simulink model "amstepsize"  (Simulink 4.00)
settings: Solver=ode45  StartTime=0.0  StopTime=1  MaxStep=.01  RelTol=1e-3
undefined symbols (not defined in the file): slcm
libraries: commanapbnd2 x1
settings Model: LastModifiedBy=agaltman  InitialStep=.01  BlockReductionOpt=off

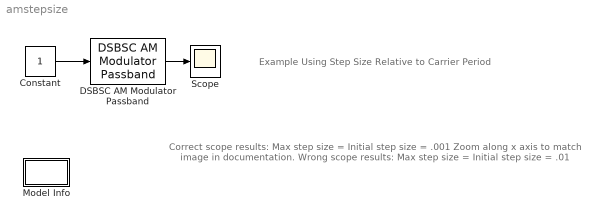
== system amstepsize ==
  note: Example Using Step Size
      | Relative to Carrier Period
  note: Correct scope results:
      | Max step size = Initial step size = .001
      | Zoom along x axis to match
      | image in documentation.
      |
      | Wrong scope results:
      | Max step size = Initial step size = .01
  Constant : Constant  Value=1
  DSBSC AM Modulator Passband : commanapbnd2/DSBSC AM Modulator Passband  Fc=100  Ph=pi/2
  Model Info : Subsystem  LoadFcn=slcm LoadBlock;  InitFcn=slcm('UpdateAllCMBlocksInThisModelInit')  mask(CMBlock){InitialSaveTempField=, InitialBlockCM=none, BlockCM=none, Frame=on, SaveTempField=, DisplayStringWithTags=Info, MaskDisplayString=Info, HorizontalTextAlignment=Center, LeftAlignmentValue=0.5, SourceBlockDiagram=amstepsize, TagMaxNumber=20, CMTag1=, CMTag2=, CMTag3=, CMTag4=, CMTag5=, CMTag6=, CMTag7=, CMTag8=, CMTag9=, CMTag10=, CMTag11=, CMTag12=, CMTag13=, CMTag14=, CMTag15=, CMTag16=, CMTag17=, CMTag18=, CMTag19=, CMTag20=}
      mask help: This block allows revision control information to be displayed within the model.
      settings: CopyFcn=slcm CopyBlock;  DeleteFcn=slcm Cancel;  PostSaveFcn=slcm('UpdateAllCMBlocksInThisModel')  NameChangeFcn=slcm Rename;  OpenFcn=commdemohelp;  RTWFcnNameOpts=Auto  RTWFileNameOpts=Auto
      mask Display: text(str2num(LeftAlignmentValue), 0.5, MaskDisplayString, 'HorizontalAlignment', HorizontalTextAlignment)
  Scope : Scope
      settings: TimeRange=auto  YMin=-5  YMax=5  SaveToWorkspace=off  SaveName=ScopeData  LimitDataPoints=on  MaxDataPoints=5000
  wires:
  Constant/1 -> DSBSC AM Modulator Passband/1
  DSBSC AM Modulator Passband/1 -> Scope/1

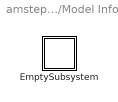
== system amstepsize/Model Info ==
  EmptySubsystem : Subsystem
      settings: RTWFcnNameOpts=Auto  RTWFileNameOpts=Auto

== system amstepsize/Model Info/EmptySubsystem ==
